simulink model "altitude_plant"  (Simulink 7.8)
settings: Solver=ode45  StartTime=0.0  StopTime=200.0  RelTol=1e-3
libraries: simulink x1
settings Model: Creator=jcotton81  LastModifiedBy=jcotton81
settings DataIOCC: LoadExternalInput=on

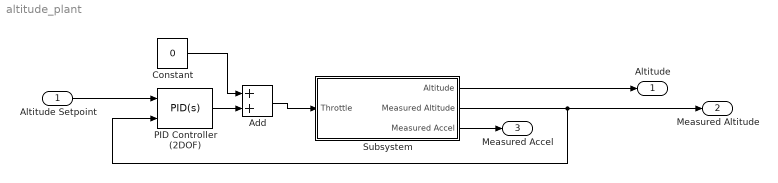
== system altitude_plant ==
  Altitude Setpoint : Inport
  Add : Sum
  Constant : Constant  Value=0
  PID Controller (2DOF) : simulink/Continuous/PID Controller (2DOF)  Controller=PID  TimeDomain=Continuous-time  SampleTime=1  IntegratorMethod=Forward Euler  FilterMethod=Forward Euler  Form=Parallel  P=0.1  I=0.0  D=0  N=100  b=1  c=1  InitialConditionSource=internal  InitialConditionForIntegrator=0  InitialConditionForFilter=0  ExternalReset=none  LimitOutput=off  UpperSaturationLimit=inf  LowerSaturationLimit=-inf  LinearizeAsGain=off  AntiWindupMode=none  Kb=1  TrackingMode=off  Kt=1  PParamMin=[]  PParamMax=[]  IParamMin=[]  IParamMax=[]  DParamMin=[]  DParamMax=[]  NParamMin=[]  NParamMax=[]  bParamMin=[]  bParamMax=[]  cParamMin=[]  cParamMax=[]  KbParamMin=[]  KbParamMax=[]  KtParamMin=[]  KtParamMax=[]  POutMin=[]  POutMax=[]  IOutMin=[]  IOutMax=[]  DOutMin=[]  DOutMax=[]  NOutMin=[]  NOutMax=[]  bOutMin=[]  bOutMax=[]  cOutMin=[]  cOutMax=[]  KbOutMin=[]  KbOutMax=[]  KtOutMin=[]  KtOutMax=[]  IntegratorOutMin=[]  IntegratorOutMax=[]  FilterOutMin=[]  FilterOutMax=[]  SumOutMin=[]  SumOutMax=[]  Sum1OutMin=[]  Sum1OutMax=[]  Sum2OutMin=[]  Sum2OutMax=[]  Sum3OutMin=[]  Sum3OutMax=[]  SumI1OutMin=[]  SumI1OutMax=[]  SumI2OutMin=[]  SumI2OutMax=[]  SumI3OutMin=[]  SumI3OutMax=[]  SumDOutMin=[]  SumDOutMax=[]  SaturationOutMin=[]  SaturationOutMax=[]  IntegratorContinuousStateAttributes=''  IntegratorStateMustResolveToSignalObject=off  IntegratorRTWStateStorageClass=Auto  FilterContinuousStateAttributes=''  FilterStateMustResolveToSignalObject=off  FilterRTWStateStorageClass=Auto
  Subsystem : Subsystem
  Altitude : Outport
  Measured Altitude : Outport  Port=2
  Measured Accel : Outport  Port=3
  wires:
  Subsystem/1(Altitude) -> Altitude/1
  Subsystem/2(Measured Altitude) -> Measured Altitude/1, PID Controller (2DOF)/2
  Subsystem/3(Measured Accel) -> Measured Accel/1
  Altitude Setpoint/1 -> PID Controller (2DOF)/1
  PID Controller (2DOF)/1 -> Add/2
  Add/1 -> Subsystem/1(Throttle)
  Constant/1 -> Add/1

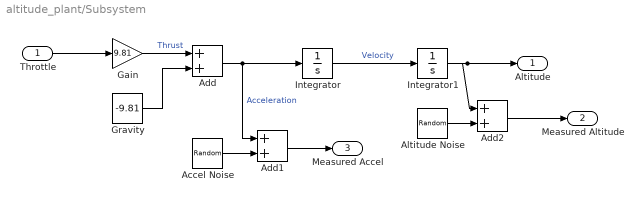
== system altitude_plant/Subsystem ==
  Throttle : Inport
  Accel Noise : RandomNumber  SampleTime=0.1
  Add : Sum
  Add1 : Sum
  Add2 : Sum
  Altitude Noise : RandomNumber  SampleTime=0.1
  Gain : Gain  Gain=9.81
  Gravity : Constant  Value=-9.81
  Integrator : Integrator
  Integrator1 : Integrator
  Altitude : Outport
  Measured Altitude : Outport  Port=2
  Measured Accel : Outport  Port=3
  wires:
  Add1/1 -> Measured Accel/1
  Altitude Noise/1 -> Add2/2
  Accel Noise/1 -> Add1/2
  Integrator1/1 -> Add2/1, Altitude/1
  Integrator/1 -> Integrator1/1  "Velocity"
  Add/1 -> Add1/1, Integrator/1  "Acceleration"
  Gravity/1 -> Add/2
  Gain/1 -> Add/1  "Thrust"
  Add2/1 -> Measured Altitude/1
  Throttle/1 -> Gain/1
